simulink model "PMSM_3"  (R2022b)
settings: Solver=VariableStepAuto  StartTime=0.0  StopTime=10.0  RelTol=1e-3
values from neighbouring files (symbols this model uses):
  Bm = 0    [param.m]
  Jm = 7.5e-6    (= 7.5e-06)    [param.m]
  Lamf = 0.1    [param.m]
  Lds = (31.07e-3)/2    (= 0.015535)    [param.m]
  Lqs = (31.07e-3)/2    (= 0.015535)    [param.m]
  p = 3    [param.m]
  Rs = 33.41/2    (= 16.705)    [param.m]
  Thetarm_Init = 0    [param.m]
  Tmax = 1.4    [param.m]
  Ts = 1/fs    (= 0.0001)    [param.m]
  Vdc = 600    [param.m]
  Wrm_Init = 0    [param.m]
undefined symbols (not defined in the file or in its folder): idVec, iqVec, Ki_id, Ki_iq, Ki_omega, Kp_id, Kp_iq, Kp_omega, LdMatrix, LqMatrix, PmMatrix, TL_fin, TL_in, Tsc, Tstep, Vnom
libraries: slpidlib x3, PMSM_lib x2, eePmsmCurrentReferenceGen x1, eeTransforms x1, eePwmGeneratorTwoLevel x1
settings Model: Creator=H290509  LastModifiedBy=H290509

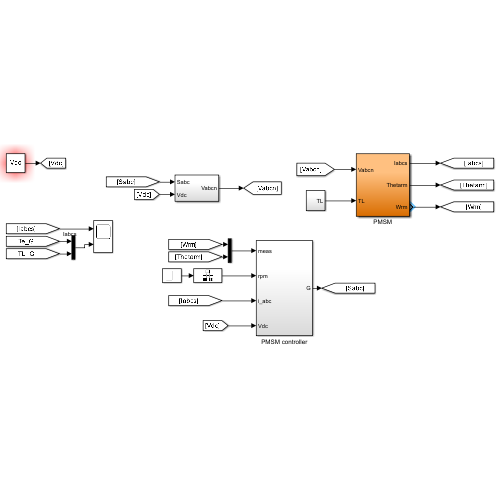
[thumbnail: Simulink's stored preview of the top-level diagram]
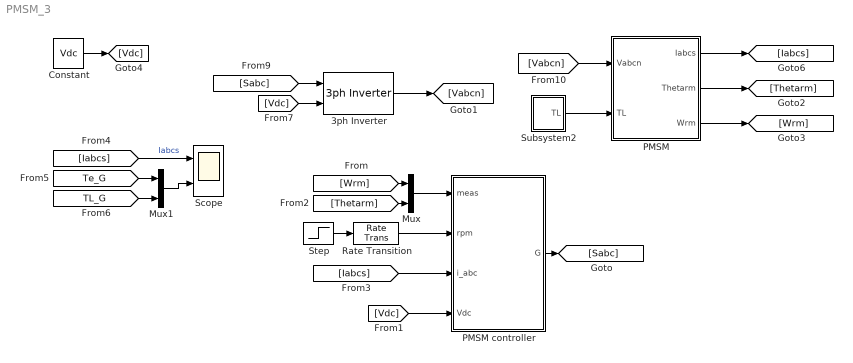
== system PMSM_3 ==
  3ph Inverter : PMSM_lib/3ph Inverter  SystemSampleTime=-1  VariantActivationTime=update diagram  Latency=0  AutoFrameSizeCalculation=off
  Constant : Constant  Value=Vdc
  Mux : Mux  Inputs=2
  Mux1 : Mux  Inputs=2
  PMSM : Subsystem
  PMSM controller : Subsystem
  Rate Transition : RateTransition
  Scope : Scope  NumInputPorts=2
  Step : Step  Time=0.03  After=1000  SampleTime=0
  Subsystem2 : Subsystem
  wires:
  PMSM/3(Wrm) -> [Wrm]
  PMSM/2(Thetarm) -> [Thetarm]
  [Sabc] -> 3ph Inverter/1
  [Vabcn] -> PMSM/1(Vabcn)
  3ph Inverter/1 -> [Vabcn]
  Subsystem2/1(TL) -> PMSM/2(TL)
  [Vdc] -> 3ph Inverter/2
  PMSM/1(Iabcs) -> [Iabcs]
  PMSM controller/1(G) -> [Sabc]
  [Vdc] -> PMSM controller/4(Vdc)
  Constant/1 -> [Vdc]
  Mux/1 -> PMSM controller/1(meas)
  [Wrm] -> Mux/1
  [Thetarm] -> Mux/2
  [Iabcs] -> PMSM controller/3(i_abc)
  Step/1 -> Rate Transition/1
  Rate Transition/1 -> PMSM controller/2(rpm)
  [Te_G] -> Mux1/1
  [Iabcs] -> Scope/1  "Iabcs"
  [TL_G] -> Mux1/2
  Mux1/1 -> Scope/2

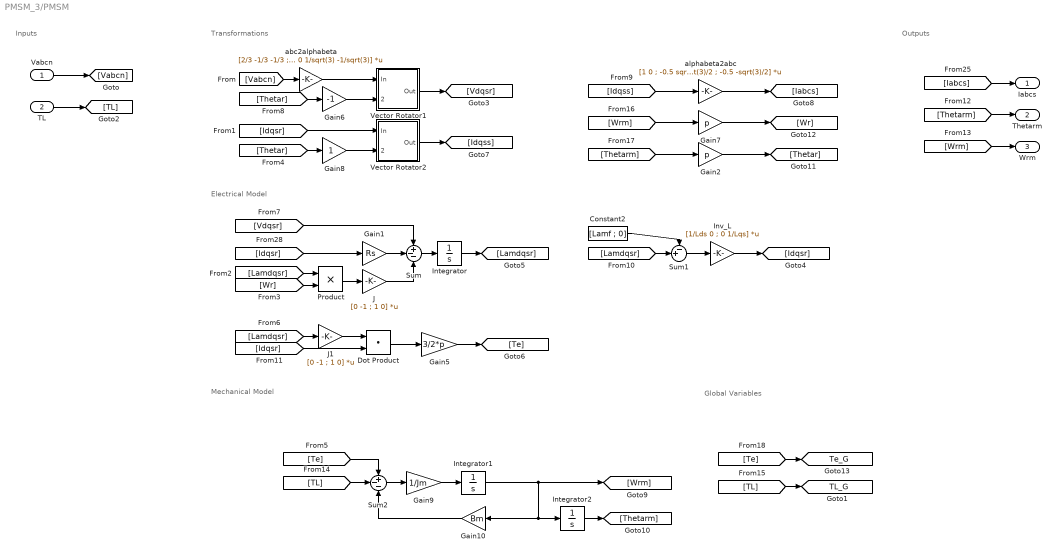
== system PMSM_3/PMSM ==
  note: Inputs
  note: Outputs
  note: Global Variables
  note: Mechanical Model
  note: Electrical Model
  note: Transformations
  Vabcn : Inport
  TL : Inport  Port=2
  Constant2 : Constant  Value=[Lamf ; 0]
  Dot Product : DotProduct  OutDataTypeStr=Inherit: Inherit via internal rule
  Gain1 : Gain  Gain=Rs
  Gain10 : Gain  Gain=Bm
  Gain2 : Gain  Gain=p
  Gain5 : Gain  Gain=3/2*p
  Gain6 : Gain  Gain=-1
  Gain7 : Gain  Gain=p
  Gain8 : Gain
  Gain9 : Gain  Gain=1/Jm
  Integrator : Integrator  InitialCondition=[Lamf ; 0]
  Integrator1 : Integrator  InitialCondition=Wrm_Init
  Integrator2 : Integrator  InitialCondition=Thetarm_Init  WrapState=on
  Inv_L : Gain  Gain=[1/Lds 0 ; 0 1/Lqs]  Multiplication=Matrix(K*u)
  J : Gain  Gain=[0 -1 ; 1 0]  Multiplication=Matrix(K*u)
  J1 : Gain  Gain=[0 -1 ; 1 0]  Multiplication=Matrix(K*u)
  Product : Product  RndMeth=Zero
  Sum : Sum  Inputs=+--
  Sum1 : Sum  Inputs=-+|
  Sum2 : Sum  Inputs=+--
  Vector Rotator1 : Subsystem
  Vector Rotator2 : Subsystem
  abc2alphabeta : Gain  Gain=[2/3 -1/3 -1/3 ; 0 1/sqrt(3) -1/sqrt(3)]  Multiplication=Matrix(K*u)  SaturateOnIntegerOverflow=on  OutDataTypeStr=Inherit: Same as input  ParamDataTypeStr=Inherit: Same as input
  alphabeta2abc : Gain  Gain=[1 0 ; -0.5 sqrt(3)/2 ; -0.5 -sqrt(3)/2]  Multiplication=Matrix(K*u)
  Iabcs : Outport
  Thetarm : Outport  Port=2
  Wrm : Outport  Port=3
  tag scope: TL_G=global, Te_G=global
  wires:
  TL/1 -> [TL]
  Vabcn/1 -> [Vabcn]
  [Te] -> [Te_G]
  [TL] -> [TL_G]
  [TL] -> Sum2/2
  [Wrm] -> Wrm/1
  Gain1/1 -> Sum/2
  J/1 -> Sum/3
  [Idqsr] -> Gain1/1
  Product/1 -> J/1
  [Wr] -> Product/2
  Sum/1 -> Integrator/1
  [Lamdqsr] -> Product/1
  [Vdqsr] -> Sum/1
  Integrator/1 -> [Lamdqsr]
  Gain5/1 -> [Te]
  [Idqsr] -> Dot Product/2
  [Lamdqsr] -> J1/1
  J1/1 -> Dot Product/1
  Dot Product/1 -> Gain5/1
  Constant2/1 -> Sum1/1
  [Lamdqsr] -> Sum1/2
  Inv_L/1 -> [Idqsr]
  Sum1/1 -> Inv_L/1
  Gain9/1 -> Integrator1/1
  Integrator1/1 -> Gain10/1, Integrator2/1, [Wrm]
  Sum2/1 -> Gain9/1
  [Te] -> Sum2/1
  Integrator2/1 -> [Thetarm]
  Gain10/1 -> Sum2/3
  Gain8/1 -> Vector Rotator2/2(Theta)
  [Thetar] -> Gain8/1
  Gain6/1 -> Vector Rotator1/2(Theta)
  [Thetar] -> Gain6/1
  Gain2/1 -> [Thetar]
  [Thetarm] -> Thetarm/1
  Vector Rotator1/1(Out) -> [Vdqsr]
  [Idqsr] -> Vector Rotator2/1(In)
  abc2alphabeta/1 -> Vector Rotator1/1(In)
  [Vabcn] -> abc2alphabeta/1
  Vector Rotator2/1(Out) -> [Idqss]
  [Idqss] -> alphabeta2abc/1
  alphabeta2abc/1 -> [Iabcs]
  Gain7/1 -> [Wr]
  [Thetarm] -> Gain2/1
  [Wrm] -> Gain7/1
  [Iabcs] -> Iabcs/1

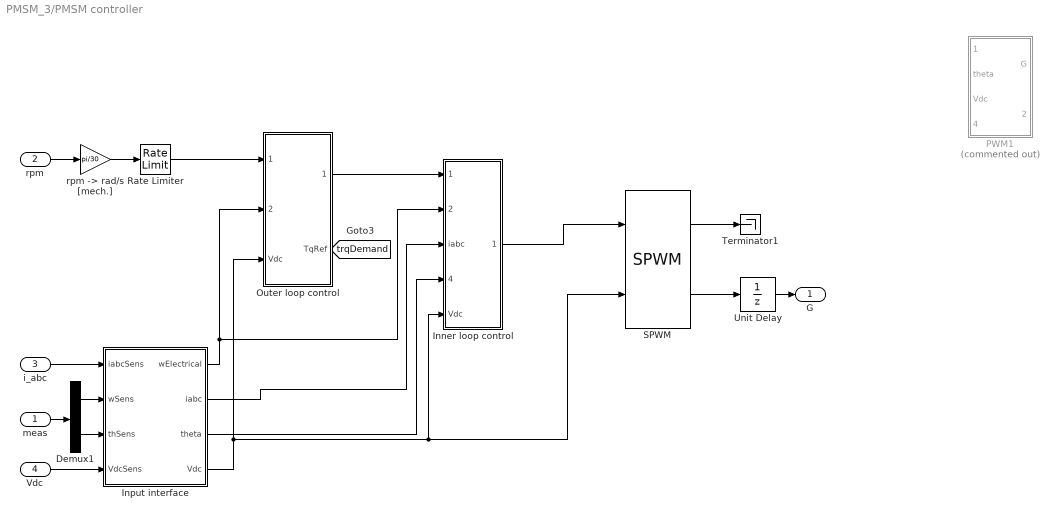
== system PMSM_3/PMSM controller ==
  meas : Inport
  rpm : Inport  Port=2
  i_abc : Inport  Port=3
  Vdc : Inport  Port=4
  Demux1 : Demux  Outputs=2
  Inner loop control : Subsystem
  Input interface : Subsystem
  Outer loop control : Subsystem
  PWM1 : Subsystem  Commented=on
  Rate Limiter : RateLimiter  RisingSlewLimit=Tmax/Jm  FallingSlewLimit=-Tmax/Jm  SampleTimeMode=inherited
  SPWM : PMSM_lib/SPWM  SystemSampleTime=-1  VariantActivationTime=update diagram  Latency=0  AutoFrameSizeCalculation=off
  Terminator1 : Terminator
  Unit Delay : UnitDelay  SampleTime=Ts  HasFrameUpgradeWarning=on
  "rpm -> rad/s [mech.]" : Gain  Gain=pi/30
  G : Outport  VectorParamsAs1DForOutWhenUnconnected=off
  tag scope: trqDemand=global
  wires:
  meas/1 -> Demux1/1
  Demux1/1 -> Input interface/2(wSens)
  rpm/1 -> "rpm -> rad/s [mech.]"/1
  "rpm -> rad/s [mech.]"/1 -> Rate Limiter/1
  SPWM/2 -> Unit Delay/1
  Input interface/1(wElectrical) -> Outer loop control/2(wElectrical), Inner loop control/2(wElectrical)
  Vdc/1 -> Input interface/4(VdcSens)
  Outer loop control/1(idqRef) -> Inner loop control/1(idq_ref)
  Rate Limiter/1 -> Outer loop control/1(Reference)
  Input interface/4(Vdc) -> SPWM/2, Inner loop control/5(Vdc), Outer loop control/3(Vdc)
  Input interface/3(theta) -> Inner loop control/4(theta)
  Inner loop control/1(vdqRef) -> SPWM/1
  Outer loop control/2(TqRef) -> [trqDemand]
  Input interface/2(iabc) -> Inner loop control/3(iabc)
  Demux1/2 -> Input interface/3(thSens)
  i_abc/1 -> Input interface/1(iabcSens)
  SPWM/1 -> Terminator1/1
  Unit Delay/1 -> G/1

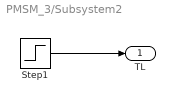
== system PMSM_3/Subsystem2 ==
  Step1 : Step  Time=Tstep  Before=TL_in  After=TL_fin
  TL : Outport
  wires:
  Step1/1 -> TL/1

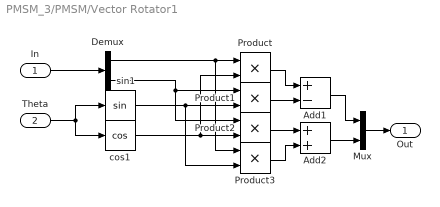
== system PMSM_3/PMSM/Vector Rotator1 ==
  In : Inport
  Theta : Inport  Port=2
  Add1 : Sum  Inputs=+-
  Add2 : Sum
  Demux : Demux  Outputs=2
  Mux : Mux  Inputs=[1 1]
  Product{,1..3} (4 alike) : Product  RndMeth=Zero
  cos1 : Trigonometry  Operator=cos
  sin1 : Trigonometry
  Out : Outport
  wires:
  Theta/1 -> cos1/1, sin1/1
  Demux/1 -> Product3/1, Product/1
  Mux/1 -> Out/1
  In/1 -> Demux/1
  Demux/2 -> Product1/1, Product2/1
  cos1/1 -> Product/2, Product2/2
  sin1/1 -> Product1/2, Product3/2
  Product/1 -> Add1/1
  Product1/1 -> Add1/2
  Add1/1 -> Mux/1
  Product2/1 -> Add2/1
  Product3/1 -> Add2/2
  Add2/1 -> Mux/2

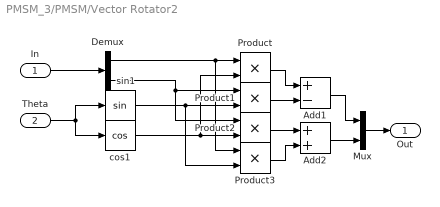
== system PMSM_3/PMSM/Vector Rotator2 ==
  In : Inport
  Theta : Inport  Port=2
  Add1 : Sum  Inputs=+-
  Add2 : Sum
  Demux : Demux  Outputs=2
  Mux : Mux  Inputs=[1 1]
  Product{,1..3} (4 alike) : Product  RndMeth=Zero
  cos1 : Trigonometry  Operator=cos
  sin1 : Trigonometry
  Out : Outport
  wires:
  Add2/1 -> Mux/2
  Product3/1 -> Add2/2
  Product2/1 -> Add2/1
  Add1/1 -> Mux/1
  Product1/1 -> Add1/2
  Product/1 -> Add1/1
  sin1/1 -> Product3/2, Product1/2
  cos1/1 -> Product2/2, Product/2
  Demux/2 -> Product2/1, Product1/1
  In/1 -> Demux/1
  Mux/1 -> Out/1
  Demux/1 -> Product/1, Product3/1
  Theta/1 -> sin1/1, cos1/1

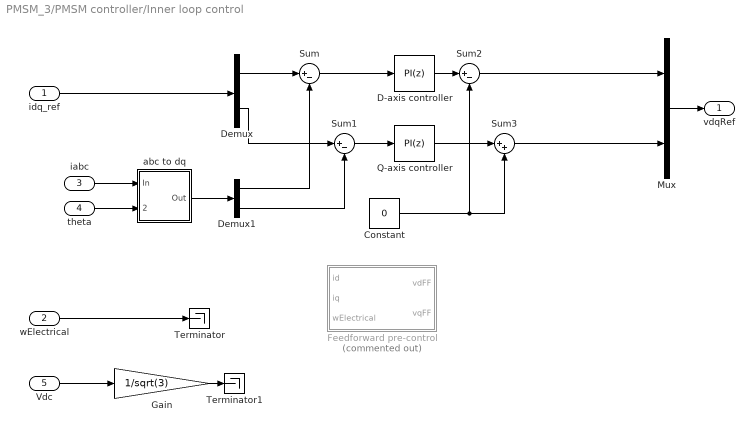
== system PMSM_3/PMSM controller/Inner loop control ==
  idq_ref : Inport
  wElectrical : Inport  Port=2
  iabc : Inport  Port=3
  theta : Inport  Port=4
  Vdc : Inport  Port=5
  Constant : Constant  Value=0
  D-axis controller : slpidlib/PID Controller  Controller=PI  Form=Parallel  TimeDomain=Discrete-time  UseExternalTs=off  SampleTime=Ts  IntegratorMethod=Forward Euler  FilterMethod=Forward Euler  ControllerParametersSource=internal  P=Kp_id  I=Ki_id  UseKiTs=off  D=0  N=100  UseFilter=on  TunerSelectOption=Transfer Function Based (PID Tuner App)  InitialConditionSource=internal  InitialConditionForIntegrator=0  InitialConditionForFilter=0  DifferentiatorICPrevScaledInput=0  ExternalReset=none  TrackingMode=off  Kt=1  LimitOutput=on  SatLimitsSource=internal  UpperSaturationLimit=Vnom/sqrt(3)  LowerSaturationLimit=-Vnom/sqrt(3)  LinearizeAsGain=on  AntiWindupMode=back-calculation  Kb=1000  LimitIntegrator=off  UpperIntegratorSaturationLimit=inf  LowerIntegratorSaturationLimit=-inf  POutMin=[]  POutMax=[]  IOutMin=[]  IOutMax=[]  DOutMin=[]  DOutMax=[]  NOutMin=[]  NOutMax=[]  SumOutMin=[]  SumOutMax=[]  SaturationOutMin=[]  SaturationOutMax=[]  PParamMin=[]  PParamMax=[]  IParamMin=[]  IParamMax=[]  DParamMin=[]  DParamMax=[]  NParamMin=[]  NParamMax=[]  KbParamMin=[]  KbParamMax=[]  KtParamMin=[]  KtParamMax=[]  KbOutMin=[]  KbOutMax=[]  KtOutMin=[]  KtOutMax=[]  IntegratorOutMin=[]  IntegratorOutMax=[]  FilterOutMin=[]  FilterOutMax=[]  SumI1OutMin=[]  SumI1OutMax=[]  SumI2OutMin=[]  SumI2OutMax=[]  SumI3OutMin=[]  SumI3OutMax=[]  SumI4OutMin=[]  SumI4OutMax=[]  SumDOutMin=[]  SumDOutMax=[]  DifferentiatorOutMin=[]  DifferentiatorOutMax=[]  FilterDiffOutCoefMin=[]  FilterDiffOutCoefMax=[]  ReciprocalOutMin=[]  ReciprocalOutMax=[]  SumDenOutMin=[]  SumDenOutMax=[]  SumNumOutMin=[]  SumNumOutMax=[]  DivideOutMin=[]  DivideOutMax=[]  UdiffTsProdOutMin=[]  UdiffTsProdOutMax=[]  NTsProdOutMin=[]  NTsProdOutMax=[]  UintegralTsProdOutMin=[]  UintegralTsProdOutMax=[]  UngainTsProdOutMin=[]  UngainTsProdOutMax=[]  ClampingZeroOutDataTypeStr=Inherit: Inherit via back propagation  ClampingZeroOutMin=[]  ClampingZeroOutMax=[]  FilterDenConstantOutDataTypeStr=Inherit: Inherit via back propagation  FilterDenConstantOutMin=[]  FilterDenConstantOutMax=[]  PCopyOutDataTypeStr=Inherit: Inherit via back propagation  PCopyOutMin=[]  PCopyOutMax=[]  NCopyOutDataTypeStr=Inherit: Inherit via back propagation  NCopyOutMin=[]  NCopyOutMax=[]  IntegratorContinuousStateAttributes=''  IntegratorStateMustResolveToSignalObject=off  IntegratorRTWStateStorageClass=Auto  FilterContinuousStateAttributes=''  FilterStateMustResolveToSignalObject=off  FilterRTWStateStorageClass=Auto  ParallelPVariant=InternalParameters  IdealPVariant=Disabled  IVariant=InternalParameters  DVariant=Disabled  IntegratorVariant=Discrete  SatVariant=Enabled  AWVariant=BackCalculation  PCopyVariant=Disabled  TRVariant=Disabled  FdbkBlocksVariant=Forward  IdealPFdbkVariant=Disabled  SatFdbkVariant=Disabled  DerivativeFilterVariant=Disabled  NVariant=Disabled  NCopyVariant=Disabled_SignalSpec  FilterICVariant=Disabled  IntegratorICVariant=InternalICs  ExternalResetVariant=Disabled  TRSumVariant=Passthrough  SumFdbkVariant=Disabled  SumVariant=Sum_PI  TsampFilterVariant=InternalTs  TsampNgainVariant=Passthrough  TsampIntegralVariant=Passthrough  ExternalSaturationOutDataTypeStr=Inherit: Same as second input
  Demux : Demux  Outputs=2
  Demux1 : Demux  Outputs=2
  Feedforward pre-control : Subsystem  Commented=on
  Gain : Gain  Gain=1/sqrt(3)
  Mux : Mux  Inputs=2
  Q-axis controller : slpidlib/PID Controller  Controller=PI  Form=Parallel  TimeDomain=Discrete-time  UseExternalTs=off  SampleTime=Ts  IntegratorMethod=Forward Euler  FilterMethod=Forward Euler  ControllerParametersSource=internal  P=Kp_iq  I=Ki_iq  UseKiTs=off  D=0  N=100  UseFilter=on  TunerSelectOption=Transfer Function Based (PID Tuner App)  InitialConditionSource=internal  InitialConditionForIntegrator=0  InitialConditionForFilter=0  DifferentiatorICPrevScaledInput=0  ExternalReset=none  TrackingMode=off  Kt=1  LimitOutput=on  SatLimitsSource=internal  UpperSaturationLimit=Vnom/sqrt(3)  LowerSaturationLimit=-Vnom/sqrt(3)  LinearizeAsGain=on  AntiWindupMode=back-calculation  Kb=1000  LimitIntegrator=off  UpperIntegratorSaturationLimit=inf  LowerIntegratorSaturationLimit=-inf  POutMin=[]  POutMax=[]  IOutMin=[]  IOutMax=[]  DOutMin=[]  DOutMax=[]  NOutMin=[]  NOutMax=[]  SumOutMin=[]  SumOutMax=[]  SaturationOutMin=[]  SaturationOutMax=[]  PParamMin=[]  PParamMax=[]  IParamMin=[]  IParamMax=[]  DParamMin=[]  DParamMax=[]  NParamMin=[]  NParamMax=[]  KbParamMin=[]  KbParamMax=[]  KtParamMin=[]  KtParamMax=[]  KbOutMin=[]  KbOutMax=[]  KtOutMin=[]  KtOutMax=[]  IntegratorOutMin=[]  IntegratorOutMax=[]  FilterOutMin=[]  FilterOutMax=[]  SumI1OutMin=[]  SumI1OutMax=[]  SumI2OutMin=[]  SumI2OutMax=[]  SumI3OutMin=[]  SumI3OutMax=[]  SumI4OutMin=[]  SumI4OutMax=[]  SumDOutMin=[]  SumDOutMax=[]  DifferentiatorOutMin=[]  DifferentiatorOutMax=[]  FilterDiffOutCoefMin=[]  FilterDiffOutCoefMax=[]  ReciprocalOutMin=[]  ReciprocalOutMax=[]  SumDenOutMin=[]  SumDenOutMax=[]  SumNumOutMin=[]  SumNumOutMax=[]  DivideOutMin=[]  DivideOutMax=[]  UdiffTsProdOutMin=[]  UdiffTsProdOutMax=[]  NTsProdOutMin=[]  NTsProdOutMax=[]  UintegralTsProdOutMin=[]  UintegralTsProdOutMax=[]  UngainTsProdOutMin=[]  UngainTsProdOutMax=[]  ClampingZeroOutDataTypeStr=Inherit: Inherit via back propagation  ClampingZeroOutMin=[]  ClampingZeroOutMax=[]  FilterDenConstantOutDataTypeStr=Inherit: Inherit via back propagation  FilterDenConstantOutMin=[]  FilterDenConstantOutMax=[]  PCopyOutDataTypeStr=Inherit: Inherit via back propagation  PCopyOutMin=[]  PCopyOutMax=[]  NCopyOutDataTypeStr=Inherit: Inherit via back propagation  NCopyOutMin=[]  NCopyOutMax=[]  IntegratorContinuousStateAttributes=''  IntegratorStateMustResolveToSignalObject=off  IntegratorRTWStateStorageClass=Auto  FilterContinuousStateAttributes=''  FilterStateMustResolveToSignalObject=off  FilterRTWStateStorageClass=Auto  ParallelPVariant=InternalParameters  IdealPVariant=Disabled  IVariant=InternalParameters  DVariant=Disabled  IntegratorVariant=Discrete  SatVariant=Enabled  AWVariant=BackCalculation  PCopyVariant=Disabled  TRVariant=Disabled  FdbkBlocksVariant=Forward  IdealPFdbkVariant=Disabled  SatFdbkVariant=Disabled  DerivativeFilterVariant=Disabled  NVariant=Disabled  NCopyVariant=Disabled_SignalSpec  FilterICVariant=Disabled  IntegratorICVariant=InternalICs  ExternalResetVariant=Disabled  TRSumVariant=Passthrough  SumFdbkVariant=Disabled  SumVariant=Sum_PI  TsampFilterVariant=InternalTs  TsampNgainVariant=Passthrough  TsampIntegralVariant=Passthrough  ExternalSaturationOutDataTypeStr=Inherit: Same as second input
  Sum : Sum  Inputs=|+-
  Sum1 : Sum  Inputs=|+-
  Sum2 : Sum  Inputs=|+-
  Sum3 : Sum  Inputs=|++
  Terminator : Terminator
  Terminator1 : Terminator
  abc to dq : Subsystem
  vdqRef : Outport  VectorParamsAs1DForOutWhenUnconnected=off
  wires:
  Vdc/1 -> Gain/1
  theta/1 -> abc to dq/2(Theta)
  iabc/1 -> abc to dq/1(In)
  Demux/1 -> Sum/1
  D-axis controller/1 -> Sum2/1
  Demux1/1 -> Sum/2
  Demux/2 -> Sum1/1
  idq_ref/1 -> Demux/1
  Q-axis controller/1 -> Sum3/1
  Sum3/1 -> Mux/2
  Sum2/1 -> Mux/1
  abc to dq/1(Out) -> Demux1/1
  Mux/1 -> vdqRef/1
  Demux1/2 -> Sum1/2
  Sum/1 -> D-axis controller/1
  Sum1/1 -> Q-axis controller/1
  wElectrical/1 -> Terminator/1
  Constant/1 -> Sum2/2, Sum3/2
  Gain/1 -> Terminator1/1

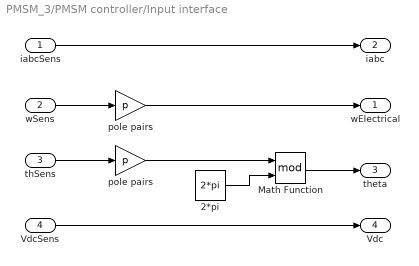
== system PMSM_3/PMSM controller/Input interface ==
  iabcSens : Inport
  wSens : Inport  Port=2
  thSens : Inport  Port=3
  VdcSens : Inport  Port=4
  2*pi : Constant  Value=2*pi  SampleTime=Ts
  Math Function : Math  Operator=mod  SignedPower=on
  pole pairs : Gain  Gain=p
  "pole pairs " : Gain  Gain=p
  wElectrical : Outport  VectorParamsAs1DForOutWhenUnconnected=off
  iabc : Outport  Port=2  VectorParamsAs1DForOutWhenUnconnected=off
  theta : Outport  Port=3  VectorParamsAs1DForOutWhenUnconnected=off
  Vdc : Outport  Port=4  VectorParamsAs1DForOutWhenUnconnected=off
  wires:
  Math Function/1 -> theta/1
  2*pi/1 -> Math Function/2
  "pole pairs "/1 -> Math Function/1
  iabcSens/1 -> iabc/1
  wSens/1 -> pole pairs/1
  thSens/1 -> "pole pairs "/1
  pole pairs/1 -> wElectrical/1
  VdcSens/1 -> Vdc/1

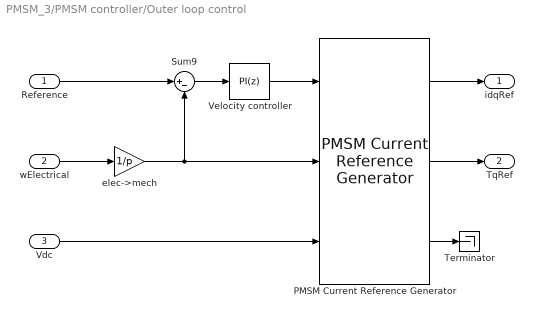
== system PMSM_3/PMSM controller/Outer loop control ==
  Reference : Inport
  wElectrical : Inport  Port=2
  Vdc : Inport  Port=3
  PMSM Current Reference Generator : eePmsmCurrentReferenceGen/PMSM Current Reference Generator  Vnom=Vnom  Pmax=Pmax  Tmax=Tmax  Ts=Tsc  RefType=Zero d-axis control  rpmVec=rpmVec  TqVec=TqVec  VdcVec=VdcVec  PWMMode=SVM: space vector modulation  ModFactor=1  idMatrix=idMatrix  iqMatrix=iqMatrix  p=p  psim=psim  Ld=Ld  Lq=Lq  Rs=Rs  RefExpEnable=0
  Sum9 : Sum  Inputs=|+-
  Terminator : Terminator
  Velocity controller : slpidlib/PID Controller  Controller=PI  Form=Parallel  TimeDomain=Discrete-time  UseExternalTs=off  SampleTime=Ts  IntegratorMethod=Forward Euler  FilterMethod=Forward Euler  ControllerParametersSource=internal  P=Kp_omega  I=Ki_omega  UseKiTs=off  D=0  N=100  UseFilter=on  TunerSelectOption=Transfer Function Based (PID Tuner App)  InitialConditionSource=internal  InitialConditionForIntegrator=0  InitialConditionForFilter=0  DifferentiatorICPrevScaledInput=0  ExternalReset=none  TrackingMode=off  Kt=1  LimitOutput=on  SatLimitsSource=internal  UpperSaturationLimit=Tmax  LowerSaturationLimit=-Tmax  LinearizeAsGain=on  AntiWindupMode=back-calculation  Kb=1000  LimitIntegrator=off  UpperIntegratorSaturationLimit=inf  LowerIntegratorSaturationLimit=-inf  POutMin=[]  POutMax=[]  IOutMin=[]  IOutMax=[]  DOutMin=[]  DOutMax=[]  NOutMin=[]  NOutMax=[]  SumOutMin=[]  SumOutMax=[]  SaturationOutMin=[]  SaturationOutMax=[]  PParamMin=[]  PParamMax=[]  IParamMin=[]  IParamMax=[]  DParamMin=[]  DParamMax=[]  NParamMin=[]  NParamMax=[]  KbParamMin=[]  KbParamMax=[]  KtParamMin=[]  KtParamMax=[]  KbOutMin=[]  KbOutMax=[]  KtOutMin=[]  KtOutMax=[]  IntegratorOutMin=[]  IntegratorOutMax=[]  FilterOutMin=[]  FilterOutMax=[]  SumI1OutMin=[]  SumI1OutMax=[]  SumI2OutMin=[]  SumI2OutMax=[]  SumI3OutMin=[]  SumI3OutMax=[]  SumI4OutMin=[]  SumI4OutMax=[]  SumDOutMin=[]  SumDOutMax=[]  DifferentiatorOutMin=[]  DifferentiatorOutMax=[]  FilterDiffOutCoefMin=[]  FilterDiffOutCoefMax=[]  ReciprocalOutMin=[]  ReciprocalOutMax=[]  SumDenOutMin=[]  SumDenOutMax=[]  SumNumOutMin=[]  SumNumOutMax=[]  DivideOutMin=[]  DivideOutMax=[]  UdiffTsProdOutMin=[]  UdiffTsProdOutMax=[]  NTsProdOutMin=[]  NTsProdOutMax=[]  UintegralTsProdOutMin=[]  UintegralTsProdOutMax=[]  UngainTsProdOutMin=[]  UngainTsProdOutMax=[]  ClampingZeroOutDataTypeStr=Inherit: Inherit via back propagation  ClampingZeroOutMin=[]  ClampingZeroOutMax=[]  FilterDenConstantOutDataTypeStr=Inherit: Inherit via back propagation  FilterDenConstantOutMin=[]  FilterDenConstantOutMax=[]  PCopyOutDataTypeStr=Inherit: Inherit via back propagation  PCopyOutMin=[]  PCopyOutMax=[]  NCopyOutDataTypeStr=Inherit: Inherit via back propagation  NCopyOutMin=[]  NCopyOutMax=[]  IntegratorContinuousStateAttributes=''  IntegratorStateMustResolveToSignalObject=off  IntegratorRTWStateStorageClass=Auto  FilterContinuousStateAttributes=''  FilterStateMustResolveToSignalObject=off  FilterRTWStateStorageClass=Auto  ParallelPVariant=InternalParameters  IdealPVariant=Disabled  IVariant=InternalParameters  DVariant=Disabled  IntegratorVariant=Discrete  SatVariant=Enabled  AWVariant=BackCalculation  PCopyVariant=Disabled  TRVariant=Disabled  FdbkBlocksVariant=Forward  IdealPFdbkVariant=Disabled  SatFdbkVariant=Disabled  DerivativeFilterVariant=Disabled  NVariant=Disabled  NCopyVariant=Disabled_SignalSpec  FilterICVariant=Disabled  IntegratorICVariant=InternalICs  ExternalResetVariant=Disabled  TRSumVariant=Passthrough  SumFdbkVariant=Disabled  SumVariant=Sum_PI  TsampFilterVariant=InternalTs  TsampNgainVariant=Passthrough  TsampIntegralVariant=Passthrough  ExternalSaturationOutDataTypeStr=Inherit: Same as second input
  elec->mech : Gain  Gain=1/p
  idqRef : Outport  VectorParamsAs1DForOutWhenUnconnected=off
  TqRef : Outport  Port=2  VectorParamsAs1DForOutWhenUnconnected=off
  wires:
  elec->mech/1 -> Sum9/2, PMSM Current Reference Generator/2
  PMSM Current Reference Generator/2 -> TqRef/1
  PMSM Current Reference Generator/1 -> idqRef/1
  Vdc/1 -> PMSM Current Reference Generator/3
  wElectrical/1 -> elec->mech/1
  Reference/1 -> Sum9/1
  Sum9/1 -> Velocity controller/1
  Velocity controller/1 -> PMSM Current Reference Generator/1
  PMSM Current Reference Generator/3 -> Terminator/1

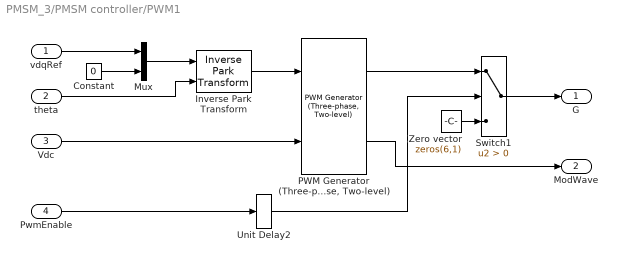
== system PMSM_3/PMSM controller/PWM1 ==
  vdqRef : Inport
  theta : Inport  Port=2
  Vdc : Inport  Port=3
  PwmEnable : Inport  Port=4
  Constant : Constant  Value=0  SampleTime=Tsc
  Inverse Park Transform : eeTransforms/Inverse Park Transform  AxisAlignment=Q-axis  PowerInvariant=off
  Mux : Mux  Inputs=2
  "PWM Generator (Three-phase, Two-level)" : eePwmGeneratorTwoLevel/PWM Generator (Three-phase, Two-level)  PWMMode=Continuous PWM (CPWM)  CPWMMode=SVM: space vector modulation  DPWMMode=60 DPWM: 60 degree discontinuous PWM  fsw=fsw  Ts=Ts
  Switch1 : Switch  Criteria=u2 > Threshold  SaturateOnIntegerOverflow=off  InputSameDT=off
  Unit Delay2 : RateTransition  OutPortSampleTime=5e-06
  Zero vector : Constant  Value=zeros(6,1)  SampleTime=Ts
  G : Outport  VectorParamsAs1DForOutWhenUnconnected=off
  ModWave : Outport  Port=2  SampleTime=Tsc  VectorParamsAs1DForOutWhenUnconnected=off
  wires:
  theta/1 -> Inverse Park Transform/2
  vdqRef/1 -> Mux/1
  Mux/1 -> Inverse Park Transform/1
  Constant/1 -> Mux/2
  "PWM Generator (Three-phase, Two-level)"/2 -> ModWave/1
  "PWM Generator (Three-phase, Two-level)"/1 -> Switch1/1
  PwmEnable/1 -> Unit Delay2/1
  Zero vector/1 -> Switch1/3
  Switch1/1 -> G/1
  Inverse Park Transform/1 -> "PWM Generator (Three-phase, Two-level)"/1
  Vdc/1 -> "PWM Generator (Three-phase, Two-level)"/2
  Unit Delay2/1 -> Switch1/2

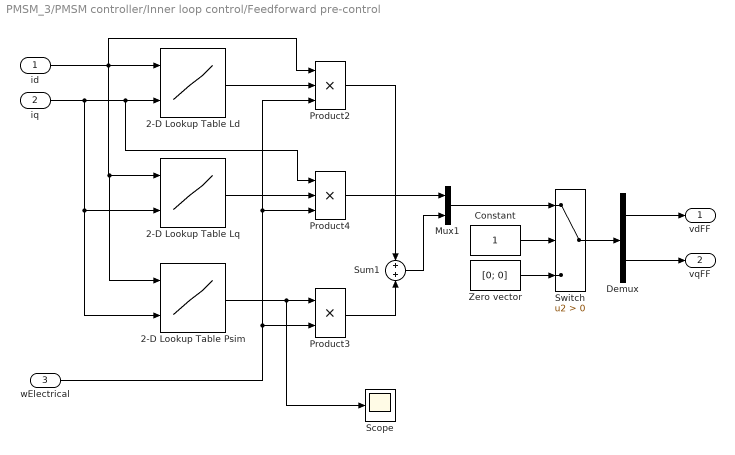
== system PMSM_3/PMSM controller/Inner loop control/Feedforward pre-control ==
  id : Inport
  iq : Inport  Port=2
  wElectrical : Inport  Port=3
  2-D Lookup Table Ld : Lookup_n-D  BreakpointsForDimension1=idVec  BreakpointsForDimension2=iqVec  Table=LdMatrix  ExtrapMethod=Clip  UseLastTableValue=on  InternalRulePriority=Speed  RndMeth=Simplest
      settings: InputPortMap=u0,u1
  2-D Lookup Table Lq : Lookup_n-D  BreakpointsForDimension1=idVec  BreakpointsForDimension2=iqVec  Table=LqMatrix  ExtrapMethod=Clip  InternalRulePriority=Speed  RndMeth=Simplest
      settings: InputPortMap=u0,u1
  2-D Lookup Table Psim : Lookup_n-D  BreakpointsForDimension1=idVec  BreakpointsForDimension2=iqVec  Table=PmMatrix  ExtrapMethod=Clip  InternalRulePriority=Speed  RndMeth=Simplest
      settings: InputPortMap=u0,u1
  Constant : Constant  SampleTime=Tsc
  Demux : Demux  Outputs=2
  Mux1 : Mux  Inputs=2
  Product2 : Product  Inputs=3
  Product3 : Product
  Product4 : Product  Inputs=3
  Scope : Scope
  Sum1 : Sum
  Switch : Switch  Criteria=u2 > Threshold  SaturateOnIntegerOverflow=off  InputSameDT=off
  Zero vector : Constant  Value=[0; 0]  SampleTime=Tsc
  vdFF : Outport  VectorParamsAs1DForOutWhenUnconnected=off
  vqFF : Outport  Port=2  VectorParamsAs1DForOutWhenUnconnected=off
  wires:
  Product3/1 -> Sum1/2
  2-D Lookup Table Lq/1 -> Product4/2
  Constant/1 -> Switch/2
  Switch/1 -> Demux/1
  Demux/1 -> vdFF/1
  Demux/2 -> vqFF/1
  2-D Lookup Table Psim/1 -> Scope/1, Product3/1
  Zero vector/1 -> Switch/3
  Sum1/1 -> Mux1/2
  2-D Lookup Table Ld/1 -> Product2/2
  iq/1 -> Product4/1, 2-D Lookup Table Ld/2, 2-D Lookup Table Lq/2, 2-D Lookup Table Psim/2
  id/1 -> Product2/1, 2-D Lookup Table Psim/1, 2-D Lookup Table Lq/1, 2-D Lookup Table Ld/1
  Product4/1 -> Mux1/1
  Mux1/1 -> Switch/1
  wElectrical/1 -> Product3/2, Product4/3, Product2/3
  Product2/1 -> Sum1/1

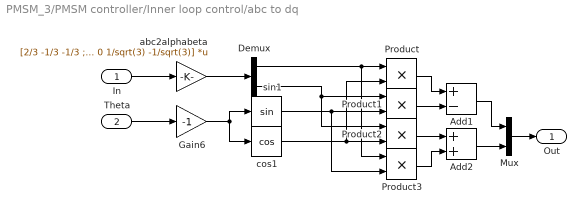
== system PMSM_3/PMSM controller/Inner loop control/abc to dq ==
  In : Inport
  Theta : Inport  Port=2
  Add1 : Sum  Inputs=+-
  Add2 : Sum
  Demux : Demux  Outputs=2
  Gain6 : Gain  Gain=-1
  Mux : Mux  Inputs=[1 1]
  Product{,1..3} (4 alike) : Product  RndMeth=Zero
  abc2alphabeta : Gain  Gain=[2/3 -1/3 -1/3 ; 0 1/sqrt(3) -1/sqrt(3)]  Multiplication=Matrix(K*u)  SaturateOnIntegerOverflow=on  OutDataTypeStr=Inherit: Same as input  ParamDataTypeStr=Inherit: Same as input
  cos1 : Trigonometry  Operator=cos
  sin1 : Trigonometry
  Out : Outport
  wires:
  Demux/1 -> Product3/1, Product/1
  Mux/1 -> Out/1
  Demux/2 -> Product1/1, Product2/1
  cos1/1 -> Product/2, Product2/2
  sin1/1 -> Product1/2, Product3/2
  Product/1 -> Add1/1
  Product1/1 -> Add1/2
  Add1/1 -> Mux/1
  Product2/1 -> Add2/1
  Product3/1 -> Add2/2
  Add2/1 -> Mux/2
  Theta/1 -> Gain6/1
  abc2alphabeta/1 -> Demux/1
  In/1 -> abc2alphabeta/1
  Gain6/1 -> cos1/1, sin1/1
